simulink model "JointSpace"  (R2019b)
settings: Solver=FixedStepAuto  StartTime=0.0  StopTime=15  FixedStep=0.001  RelTol=1e-3  EnableMultiTasking=on
values from neighbouring files (symbols this model uses):
  g = 9.81    [main11.m]    (also in main12.m; main13.m; main21.m; main22.m)
  Kp = diag([1 1])    [main21.m]    (also in main22.m = diag([1 0.2]))
  Kv = diag([2 2])    [main21.m]    (also in main22.m)
  l1 = 1    [main11.m]    (also in main12.m; main13.m; main21.m; main22.m)
  l2 = 1    [main11.m]    (also in main12.m; main13.m; main21.m; main22.m)
  m1 = 1    [main11.m]    (also in main12.m; main13.m; main21.m; main22.m)
  m2 = 1    [main11.m]    (also in main12.m; main13.m; main21.m; main22.m)
  q_d = [0; pi/2]    [main21.m]    (also in main22.m)
  x_init = [0;0;0;0]    [main11.m]    (also in main12.m = [0;pi/2;0;0]; main13.m; main21.m = [-pi/2;0;0;0]; main22.m = [-pi/2;0;0;0])
undefined symbols (not defined in the file or in its folder): x
libraries: dspinverses x1
settings Model: Creator=Sondre  LastModifiedBy=Neets
settings DataIOCC: ReturnWorkspaceOutputs=off
settings OptimizationCC: LifeSpan=inf
settings DebuggingCC: SFUnexpectedBacktrackingDiag=warning  SFNoUnconditionalDefaultTransitionDiag=warning  ArithmeticOperatorsInVariantConditions=warning
settings SFSimCC: SimUseLocalCustomCode=off  CustomCodeUndefinedFunction=UseInterfaceOnly
settings RTWCC: RTWUseLocalCustomCode=off
settings CodeAppCC: StateflowObjectComments=on
settings GRTTargetCC: TargetLangStandard=C89/C90 (ANSI)  GeneratePreprocessorConditionals=Disable all
settings ConfigComp: CovMetricSettings=dw  CovHtmlReporting=on  CovSaveCumulativeToWorkspaceVar=on  CovSaveSingleToWorkspaceVar=on  CovExternalEMLEnable=off

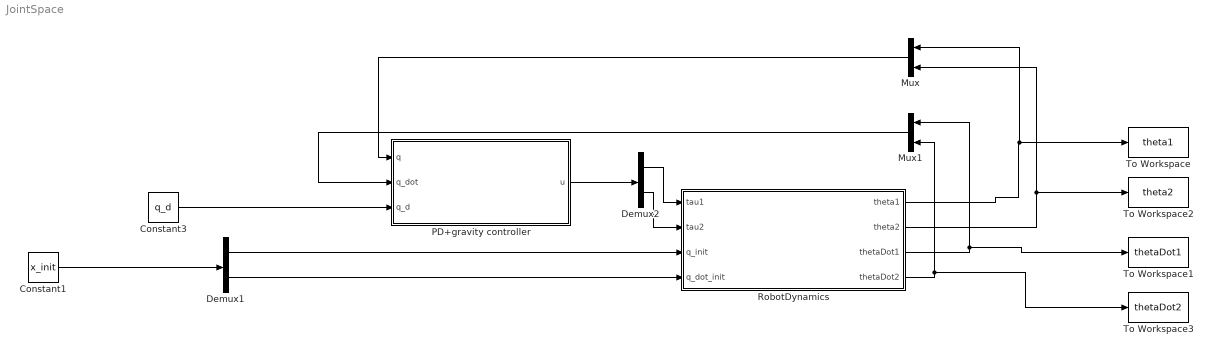
== system JointSpace ==
  Constant1 : Constant  Value=x_init
  Constant3 : Constant  Value=q_d
  Demux1 : Demux  Outputs=2
  Demux2 : Demux  Outputs=2
  Mux : Mux  Inputs=2
  Mux1 : Mux  Inputs=2
  PD+gravity controller : Subsystem
  RobotDynamics : Subsystem
  To Workspace : ToWorkspace  VariableName=theta1  SaveFormat=Timeseries  SampleTime=-1
  To Workspace1 : ToWorkspace  VariableName=thetaDot1  SaveFormat=Timeseries  SampleTime=-1
  To Workspace2 : ToWorkspace  VariableName=theta2  SaveFormat=Timeseries  SampleTime=-1
  To Workspace3 : ToWorkspace  VariableName=thetaDot2  SaveFormat=Timeseries  SampleTime=-1
  wires:
  Mux1/1 -> PD+gravity controller/2("q_dot ")
  RobotDynamics/4(thetaDot2) -> Mux1/2, To Workspace3/1
  PD+gravity controller/1("u ") -> Demux2/1
  Constant1/1 -> Demux1/1
  Mux/1 -> PD+gravity controller/1(q)
  Demux1/1 -> RobotDynamics/3(q_init)
  RobotDynamics/3(thetaDot1) -> Mux1/1, To Workspace1/1
  RobotDynamics/2(theta2) -> Mux/2, To Workspace2/1
  RobotDynamics/1(theta1) -> Mux/1, To Workspace/1
  Constant3/1 -> PD+gravity controller/3(q_d)
  Demux1/2 -> RobotDynamics/4(q_dot_init)
  Demux2/1 -> RobotDynamics/1(tau1)
  Demux2/2 -> RobotDynamics/2(tau2)

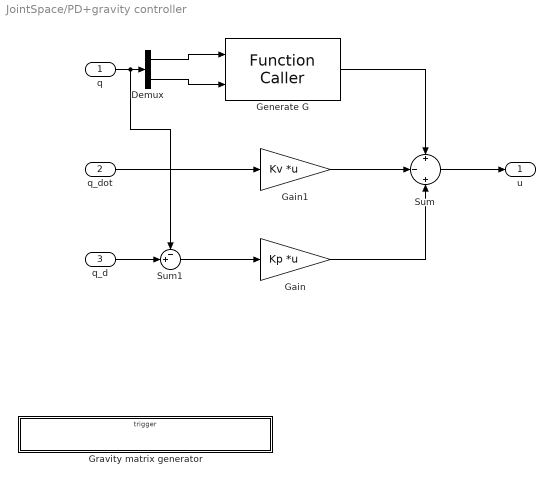
== system JointSpace/PD+gravity controller ==
  q : Inport
  "q_dot " : Inport  Port=2
  q_d : Inport  Port=3
  Demux : Demux  Outputs=2
  Gain : Gain  Gain=Kp  Multiplication=Matrix(K*u)
  Gain1 : Gain  Gain=Kv  Multiplication=Matrix(K*u)
  Generate G : FunctionCaller  FunctionPrototype=G = G(theta1,theta2)  InputArgumentSpecifications=<Enter example>  OutputArgumentSpecifications=<Enter example>
  "Gravity matrix generator " : Subsystem  TreatAsAtomicUnit=on
  Sum : Sum  Inputs=+|-|+
  Sum1 : Sum  Inputs=-+|
  "u " : Outport
  wires:
  q/1 -> Sum1/1, Demux/1
  Demux/1 -> Generate G/1
  Demux/2 -> Generate G/2
  q_d/1 -> Sum1/2
  Sum1/1 -> Gain/1
  "q_dot "/1 -> Gain1/1
  Gain1/1 -> Sum/2
  Gain/1 -> Sum/3
  Generate G/1 -> Sum/1
  Sum/1 -> "u "/1

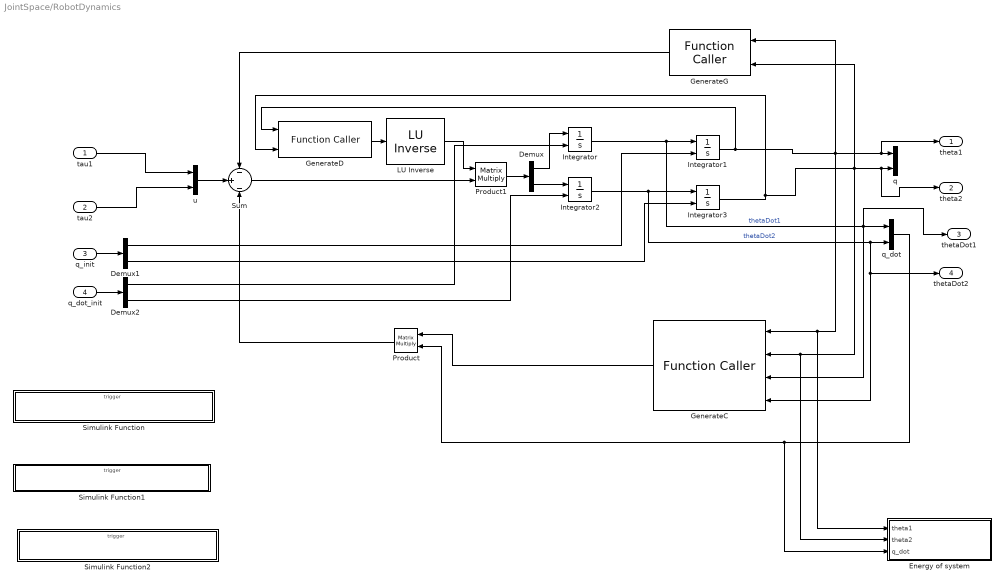
== system JointSpace/RobotDynamics ==
  tau1 : Inport
  tau2 : Inport  Port=2
  q_init : Inport  Port=3
  q_dot_init : Inport  Port=4
  " LU Inverse" : dspinverses/ LU Inverse
      settings: SourceProductName=DSP System Toolbox
  Demux : Demux  Outputs=2
  Demux1 : Demux  Outputs=2
  Demux2 : Demux  Outputs=2
  Energy of system : Subsystem
  GenerateC : FunctionCaller  FunctionPrototype=CQ = CMatrix(theta1,theta2,thetaDot1,thetaDot2)  InputArgumentSpecifications=<Enter example>  OutputArgumentSpecifications=<Enter example>
  GenerateD : FunctionCaller  FunctionPrototype=DQ = DEnergyMatrix(theta1,theta2)  InputArgumentSpecifications=<Enter example>  OutputArgumentSpecifications=<Enter example>
  GenerateG : FunctionCaller  FunctionPrototype=GQ = GravityMatrix(theta1,theta2)  InputArgumentSpecifications=<Enter example>  OutputArgumentSpecifications=<Enter example>
  Integrator : Integrator  InitialConditionSource=external
  Integrator1 : Integrator  InitialConditionSource=external
  Integrator2 : Integrator  InitialConditionSource=external  InitialCondition=x(
  Integrator3 : Integrator  InitialConditionSource=external
  Product : Product  Multiplication=Matrix(*)
  Product1 : Product  Multiplication=Matrix(*)
  Simulink Function : Subsystem  TreatAsAtomicUnit=on
  Simulink Function1 : Subsystem  TreatAsAtomicUnit=on
  Simulink Function2 : Subsystem  TreatAsAtomicUnit=on
  Sum : Sum  Inputs=-|+|-
  q : Concatenate
  q_dot : Concatenate
  u : Concatenate
  theta1 : Outport
  theta2 : Outport  Port=2
  thetaDot1 : Outport  Port=3
  thetaDot2 : Outport  Port=4
  wires:
  tau2/1 -> u/2
  tau1/1 -> u/1
  u/1 -> Sum/2
  Product/1 -> Sum/3
  GenerateG/1 -> Sum/1
  Sum/1 -> Product1/2
  GenerateC/1 -> Product/1
  GenerateD/1 -> " LU Inverse"/1
  " LU Inverse"/1 -> Product1/1
  Demux/1 -> Integrator/1
  Integrator/1 -> Integrator1/1, q_dot/1, GenerateC/3, thetaDot1/1  "thetaDot1"
  Demux/2 -> Integrator2/1
  Integrator2/1 -> GenerateC/4, thetaDot2/1, q_dot/2, Integrator3/1  "thetaDot2"
  Product1/1 -> Demux/1
  Integrator1/1 -> GenerateD/1, theta1/1, q/1, GenerateG/1, Energy of system/1(theta1), GenerateC/1
  q_init/1 -> Demux1/1
  q_dot_init/1 -> Demux2/1
  Demux2/1 -> Integrator/2
  Demux2/2 -> Integrator2/2
  Demux1/1 -> Integrator1/2
  Demux1/2 -> Integrator3/2
  Integrator3/1 -> GenerateD/2, Energy of system/2(theta2), GenerateC/2, GenerateG/2, theta2/1, q/2
  q_dot/1 -> Energy of system/3(q_dot), Product/2

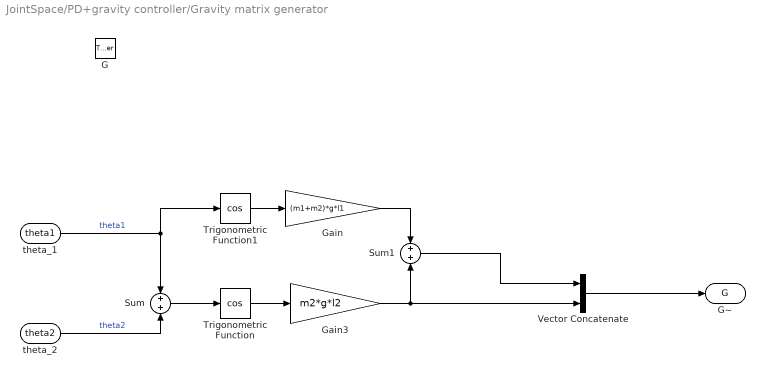
== system JointSpace/PD+gravity controller/Gravity matrix generator  ==
  G : TriggerPort  TriggerType=function-call  IsSimulinkFunction=on  FunctionName=G  FunctionVisibility=scoped  VariantControl=Variant
  Gain : Gain  Gain=(m1+m2)*g*l1
  Gain3 : Gain  Gain=m2*g*l2
  Sum : Sum  Inputs=+|+
  Sum1 : Sum  Inputs=+|+
  Trigonometric Function : Trigonometry  Operator=cos
  Trigonometric Function1 : Trigonometry  Operator=cos
  Vector Concatenate : Concatenate
  theta_1 : ArgIn  DisableCoverage=on  ArgumentName=theta1
  theta_2 : ArgIn  DisableCoverage=on  Port=2  ArgumentName=theta2
  G~ : ArgOut  DisableCoverage=on  PortDimensions=[2 1]  ArgumentName=G
  wires:
  theta_1/1 -> Trigonometric Function1/1, Sum/1  "theta1"
  theta_2/1 -> Sum/2  "theta2"
  Sum/1 -> Trigonometric Function/1
  Vector Concatenate/1 -> G~/1
  Trigonometric Function1/1 -> Gain/1
  Trigonometric Function/1 -> Gain3/1
  Gain/1 -> Sum1/1
  Gain3/1 -> Sum1/2, Vector Concatenate/2
  Sum1/1 -> Vector Concatenate/1

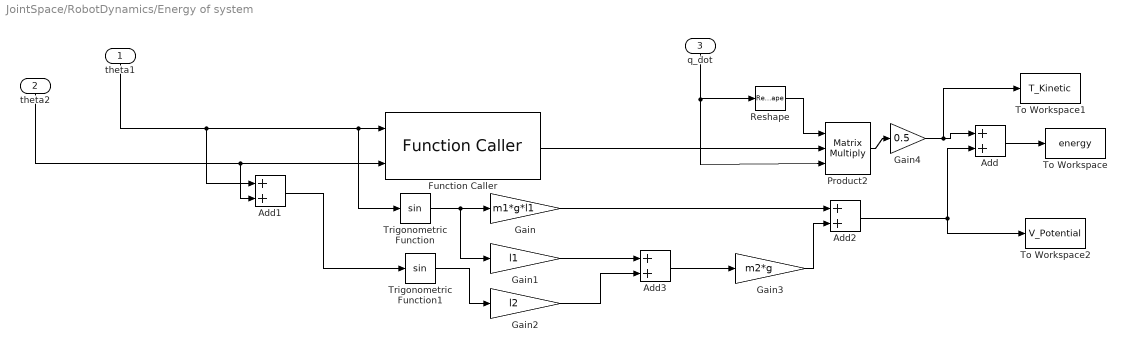
== system JointSpace/RobotDynamics/Energy of system ==
  theta1 : Inport
  theta2 : Inport  Port=2
  q_dot : Inport  Port=3
  Add{,1..3} (4 alike) : Sum
  Function Caller : FunctionCaller  FunctionPrototype=DQ = DEnergyMatrix(theta1,theta2)  InputArgumentSpecifications=<Enter example>  OutputArgumentSpecifications=<Enter example>
  Gain : Gain  Gain=m1*g*l1
  Gain1 : Gain  Gain=l1
  Gain2 : Gain  Gain=l2
  Gain3 : Gain  Gain=m2*g
  Gain4 : Gain  Gain=0.5
  Product2 : Product  Inputs=3  Multiplication=Matrix(*)
  Reshape : Reshape  OutputDimensionality=Row vector (2-D)
  To Workspace : ToWorkspace  VariableName=energy  SaveFormat=Timeseries  SampleTime=-1
  To Workspace1 : ToWorkspace  VariableName=T_Kinetic  SaveFormat=Timeseries  SampleTime=-1
  To Workspace2 : ToWorkspace  VariableName=V_Potential  SaveFormat=Timeseries  SampleTime=-1
  Trigonometric Function : Trigonometry
  Trigonometric Function1 : Trigonometry
  wires:
  theta2/1 -> Function Caller/2, Add1/2
  theta1/1 -> Function Caller/1, Trigonometric Function/1, Add1/1
  q_dot/1 -> Reshape/1, Product2/3
  Add/1 -> To Workspace/1
  Gain1/1 -> Add3/1
  Trigonometric Function/1 -> Gain1/1, Gain/1
  Trigonometric Function1/1 -> Gain2/1
  Reshape/1 -> Product2/1
  Gain4/1 -> To Workspace1/1, Add/1
  Gain/1 -> Add2/1
  Add3/1 -> Gain3/1
  Add2/1 -> Add/2, To Workspace2/1
  Gain3/1 -> Add2/2
  Add1/1 -> Trigonometric Function1/1
  Product2/1 -> Gain4/1
  Gain2/1 -> Add3/2
  Function Caller/1 -> Product2/2

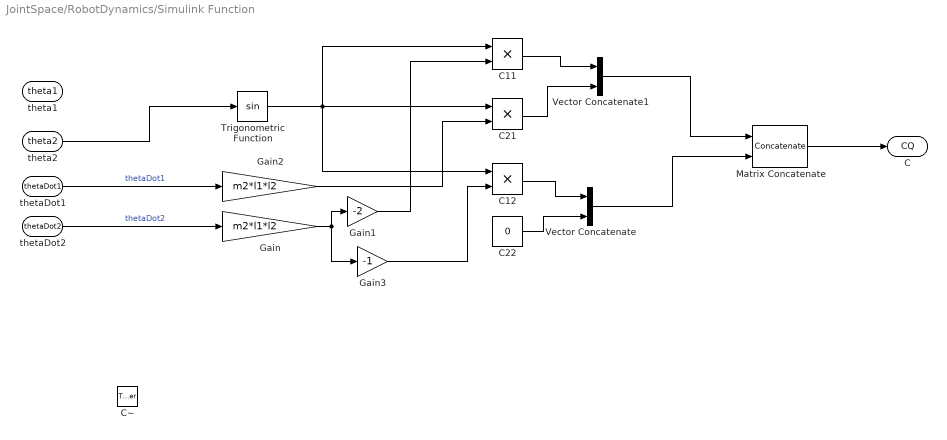
== system JointSpace/RobotDynamics/Simulink Function ==
  C~ : TriggerPort  TriggerType=function-call  IsSimulinkFunction=on  FunctionName=CMatrix  FunctionVisibility=scoped  VariantControl=Variant
  C11 : Product
  C12 : Product
  C21 : Product
  C22 : Constant  Value=0
  Gain : Gain  Gain=m2*l1*l2
  Gain1 : Gain  Gain=-2
  Gain2 : Gain  Gain=m2*l1*l2
  Gain3 : Gain  Gain=-1
  Matrix Concatenate : Concatenate  Mode=Multidimensional array  ConcatenateDimension=2
  Trigonometric Function : Trigonometry
  Vector Concatenate : Concatenate
  Vector Concatenate1 : Concatenate
  theta1 : ArgIn  DisableCoverage=on  ArgumentName=theta1
  theta2 : ArgIn  DisableCoverage=on  Port=2  ArgumentName=theta2
  thetaDot1 : ArgIn  DisableCoverage=on  Port=3  ArgumentName=thetaDot1
  thetaDot2 : ArgIn  DisableCoverage=on  Port=4  ArgumentName=thetaDot2
  C : ArgOut  DisableCoverage=on  PortDimensions=[2 2]  ArgumentName=CQ
  wires:
  thetaDot1/1 -> Gain2/1  "thetaDot1"
  thetaDot2/1 -> Gain/1  "thetaDot2"
  Trigonometric Function/1 -> C12/1, C11/1, C21/1
  C11/1 -> Vector Concatenate1/1
  Gain/1 -> Gain3/1, Gain1/1
  Gain1/1 -> C11/2
  C21/1 -> Vector Concatenate1/2
  Gain2/1 -> C21/2
  Gain3/1 -> C12/2
  C12/1 -> Vector Concatenate/1
  C22/1 -> Vector Concatenate/2
  theta2/1 -> Trigonometric Function/1
  Matrix Concatenate/1 -> C/1
  Vector Concatenate1/1 -> Matrix Concatenate/1
  Vector Concatenate/1 -> Matrix Concatenate/2

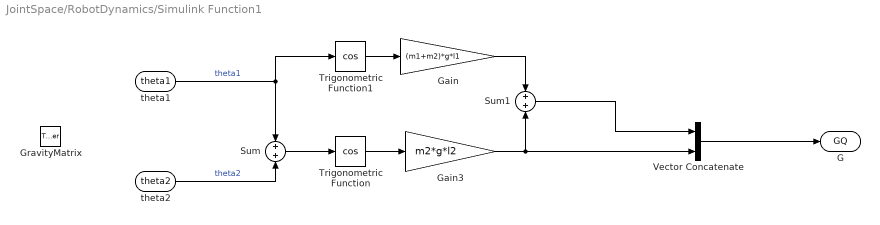
== system JointSpace/RobotDynamics/Simulink Function1 ==
  GravityMatrix : TriggerPort  TriggerType=function-call  IsSimulinkFunction=on  FunctionName=GravityMatrix  FunctionVisibility=scoped  VariantControl=Variant
  Gain : Gain  Gain=(m1+m2)*g*l1
  Gain3 : Gain  Gain=m2*g*l2
  Sum : Sum  Inputs=+|+
  Sum1 : Sum  Inputs=+|+
  Trigonometric Function : Trigonometry  Operator=cos
  Trigonometric Function1 : Trigonometry  Operator=cos
  Vector Concatenate : Concatenate
  theta1 : ArgIn  DisableCoverage=on  ArgumentName=theta1
  theta2 : ArgIn  DisableCoverage=on  Port=2  ArgumentName=theta2
  G : ArgOut  DisableCoverage=on  PortDimensions=[2 1]  ArgumentName=GQ
  wires:
  theta1/1 -> Trigonometric Function1/1, Sum/1  "theta1"
  theta2/1 -> Sum/2  "theta2"
  Sum/1 -> Trigonometric Function/1
  Vector Concatenate/1 -> G/1
  Trigonometric Function1/1 -> Gain/1
  Trigonometric Function/1 -> Gain3/1
  Gain/1 -> Sum1/1
  Gain3/1 -> Sum1/2, Vector Concatenate/2
  Sum1/1 -> Vector Concatenate/1

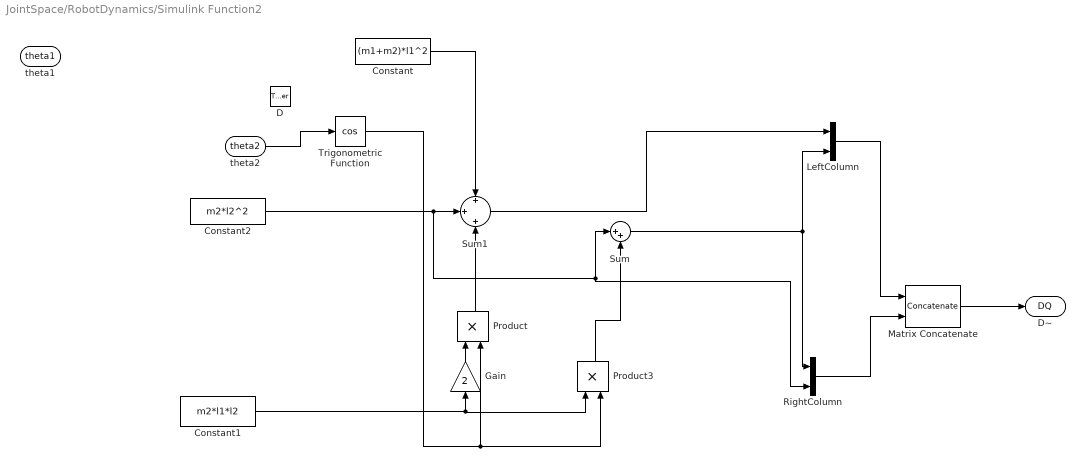
== system JointSpace/RobotDynamics/Simulink Function2 ==
  D : TriggerPort  TriggerType=function-call  IsSimulinkFunction=on  FunctionName=DEnergyMatrix  FunctionVisibility=scoped  VariantControl=Variant
  Constant : Constant  Value=(m1+m2)*l1^2
  Constant1 : Constant  Value=m2*l1*l2
  Constant2 : Constant  Value=m2*l2^2
  Gain : Gain  Gain=2
  LeftColumn : Concatenate
  Matrix Concatenate : Concatenate  Mode=Multidimensional array  ConcatenateDimension=2
  Product : Product
  Product3 : Product
  RightColumn : Concatenate
  Sum : Sum  Inputs=|++
  Sum1 : Sum  Inputs=+|+|+
  Trigonometric Function : Trigonometry  Operator=cos
  theta1 : ArgIn  DisableCoverage=on  ArgumentName=theta1
  theta2 : ArgIn  DisableCoverage=on  Port=2  ArgumentName=theta2
  D~ : ArgOut  DisableCoverage=on  PortDimensions=[2 2]  ArgumentName=DQ
  wires:
  theta2/1 -> Trigonometric Function/1
  Matrix Concatenate/1 -> D~/1
  Constant1/1 -> Product3/1, Gain/1
  Gain/1 -> Product/1
  Product/1 -> Sum1/3
  Constant/1 -> Sum1/1
  Constant2/1 -> RightColumn/2, Sum/1, Sum1/2
  Sum1/1 -> LeftColumn/1
  Product3/1 -> Sum/2
  Trigonometric Function/1 -> Product/2, Product3/2
  Sum/1 -> RightColumn/1, LeftColumn/2
  LeftColumn/1 -> Matrix Concatenate/1
  RightColumn/1 -> Matrix Concatenate/2
